simulink model "B_SinePWM_Control_Inverter"  (Simulink 8.4)
settings: Solver=ode45  StartTime=0.0  StopTime=inf  RelTol=1e-3
libraries: powerlib x10, simulink x2
settings Model: Creator=ELECTRICAL-HOD  LastModifiedBy=INTEL

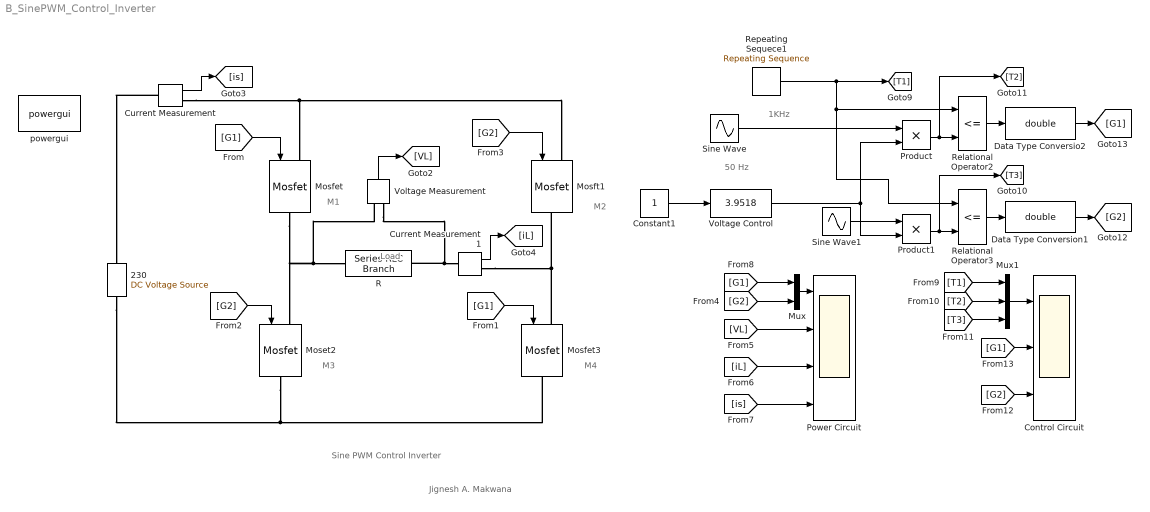
== system B_SinePWM_Control_Inverter ==
  note: Load
  note: M1
  note: M4
  note: M3
  note: M2
  note: Jignesh A. Makwana
  note: Sine PWM Control Inverter
  note: 50 Hz
  note: 1KHz
  230 : powerlib/Electrical Sources/DC Voltage Source  Amplitude=230  Measurements=None
  Constant1 : Constant
  Control Circuit : Scope  NumInputPorts=3
      settings: TimeRange=0.04  YMin=-2.5~-0.2~-0.2  YMax=5.5~1.2~1.2  MaxDataPoints=10000
  Current Measurement : powerlib/Measurements/Current Measurement  PhasorSimulation=off  OutputType=Complex  PSBequivalent=0
  Current Measurement1 : powerlib/Measurements/Current Measurement  PhasorSimulation=off  OutputType=Complex  PSBequivalent=0
  Data Type Conversio2 : DataTypeConversion  OutDataTypeStr=double
  Data Type Conversion1 : DataTypeConversion  OutDataTypeStr=double
  Moset2 : powerlib/Power Electronics/Mosfet  Ron=0.1  Lon=0  Rd=0.01  Vfd=0  IC=0  Rs=1e5  Cs=inf  Measurements=off
  Mosfet : powerlib/Power Electronics/Mosfet  Ron=0.1  Lon=0  Rd=0.01  Vfd=0  IC=0  Rs=1e5  Cs=inf  Measurements=off
  Mosfet3 : powerlib/Power Electronics/Mosfet  Ron=0.1  Lon=0  Rd=0.01  Vfd=0  IC=0  Rs=1e5  Cs=inf  Measurements=off
  Mosft1 : powerlib/Power Electronics/Mosfet  Ron=0.1  Lon=0  Rd=0.01  Vfd=0  IC=0  Rs=1e5  Cs=inf  Measurements=off
  Mux : Mux  Inputs=2
  Mux1 : Mux  Inputs=3
  Power Circuit : Scope  NumInputPorts=4
      settings: TimeRange=0.04  YMin=-0.2~-250~-0.25~1.38778e-017  YMax=5.2~250~0.25~0.25  MaxDataPoints=15000
  Product : Product  RndMeth=Zero
  Product1 : Product  RndMeth=Zero
  R : powerlib/Elements/Series RLC Branch  LConnTagsString=__new0  RConnTagsString=__new0  BranchType=R  Resistance=10  Inductance=0.1e-3  SetiL0=off  InitialCurrent=0  Capacitance=10e-6  Setx0=off  InitialVoltage=0  Measurements=None
  Relational Operator2 : RelationalOperator  Operator=<=  OutDataTypeStr=boolean
  Relational Operator3 : RelationalOperator  Operator=<=  OutDataTypeStr=boolean
  Repeating Sequece1 : simulink/Sources/Repeating Sequence  rep_seq_t=[0 0.0005 0.001]  rep_seq_y=[0.1 5.1 0.1]
  Sine Wave : Sin  Frequency=50*2*pi  SampleTime=0
  Sine Wave1 : Sin  Frequency=50*2*pi  Phase=pi  SampleTime=0
  Voltage Control : simulink/Math Operations/Slider Gain  low=0  gain=3.9518  high=5
  Voltage Measurement : powerlib/Measurements/Voltage Measurement  PhasorSimulation=off  OutputType=Complex  PSBequivalent=0
  powergui : powerlib/powergui  Priority=1  SimulationMode=Discrete  SolverType=Tustin  SampleTime=1e-6  frequency=60  SPID=off  DisableSnubberDevices=off  DisableRonSwitches=off  DisableVfSwitches=off  SwTol=0  DisplayEquations=off  Interpol=off  methode=off  Ts=0  frequencyindice=0  Pbase=100e6  ErrMax=1e-4  Iterations=50  UnitsV=kV  UnitsW=MW  FunctionMessages=off  echomessages=off  HookPort=off  EnableUseOfTLC=off  x0status=blocks  RestoreLinks=warning  ResistiveCurrentMeasurement=off  Frange=[0:2:500]  Ylog=off  Xlog=on  ShowGrid=off  save=off  variable=ZData  structure=0  ZoomFFT=off  StartTime=0.0  cycles=1  DisplayStyle=1  fundamental=60  FreqAxis=off  MaxFrequency=1000  frequencyindicesteady=1  RmsSteady=1  display=off
  wires:
  Voltage Measurement/1 -> [VL]
  Current Measurement/1 -> [is]
  Current Measurement1/1 -> [iL]
  [VL] -> Power Circuit/2
  [iL] -> Power Circuit/3
  [is] -> Power Circuit/4
  [G2] -> Mux/2
  [G1] -> Mux/1
  Mux/1 -> Power Circuit/1
  [G1] -> Mosfet3/1
  [G2] -> Mosft1/1
  [G2] -> Moset2/1
  [G1] -> Mosfet/1
  Mux1/1 -> Control Circuit/1
  [T1] -> Mux1/1
  [T2] -> Mux1/2
  [T3] -> Mux1/3
  [G1] -> Control Circuit/2
  [G2] -> Control Circuit/3
  Product/1 -> Relational Operator2/2, [T2]
  Sine Wave/1 -> Product/1
  Constant1/1 -> Voltage Control/1
  Voltage Control/1 -> Product/2, Product1/2
  Product1/1 -> Relational Operator3/2, [T3]
  Sine Wave1/1 -> Product1/1
  Data Type Conversion1/1 -> [G2]
  Data Type Conversio2/1 -> [G1]
  Relational Operator2/1 -> Data Type Conversio2/1
  Relational Operator3/1 -> Data Type Conversion1/1
  Repeating Sequece1/1 -> [T1], Relational Operator3/1, Relational Operator2/1
  connections:
  Mosfet/RConn1 -- Moset2/LConn1 -- R/LConn1 -- Voltage Measurement/LConn1
  Voltage Measurement/LConn2 -- R/RConn1 -- Current Measurement1/LConn1
  230/LConn1 -- Mosfet3/RConn1 -- Moset2/RConn1
  Current Measurement/RConn1 -- Mosft1/LConn1 -- Mosfet/LConn1
  Current Measurement/LConn1 -- 230/RConn1
  Mosfet3/LConn1 -- Mosft1/RConn1 -- Current Measurement1/RConn1
